simulink model "eomIntegratorChain"  (R2024b)
settings: Solver=ode15s  StartTime=0.0  StopTime=40  MaxStep=0.0001  RelTol=1e-6
values from neighbouring files (symbols this model uses):
  A : value not decoded    [eomParameters.sldd]
  B : value not decoded    [eomParameters.sldd]
  b = 0.1    [eomParameters.sldd]
  C : value not decoded    [eomParameters.sldd]
  D : value not decoded    [eomParameters.sldd]
  d : value not decoded    [eomParameters.sldd]
  E : value not decoded    [eomParameters.sldd]
  F : value not decoded    [eomParameters.sldd]
  H : value not decoded    [eomParameters.sldd]
  I : value not decoded    [eomParameters.sldd]
  J : value not decoded    [eomParameters.sldd]
  K : value not decoded    [eomParameters.sldd]
  L_1 : value not decoded    [eomParameters.sldd]
  mu = 0.4    [eomParameters.sldd]
  mu_r = 0.001    [eomParameters.sldd]
undefined symbols (not defined in the file or in its folder): DiscIntNeverNeededParam
settings Model: DataDictionary=eomParameters.sldd  Creator=nilgunozbulbul  LastModifiedBy=nilgunozbulbul
settings DebuggingCC: SignalInfNanChecking=error

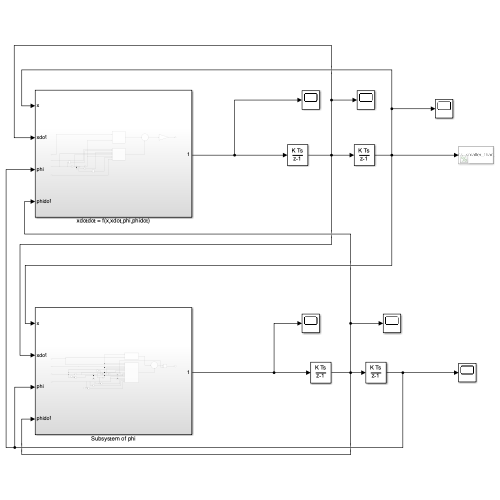
[thumbnail: Simulink's stored preview of the top-level diagram]
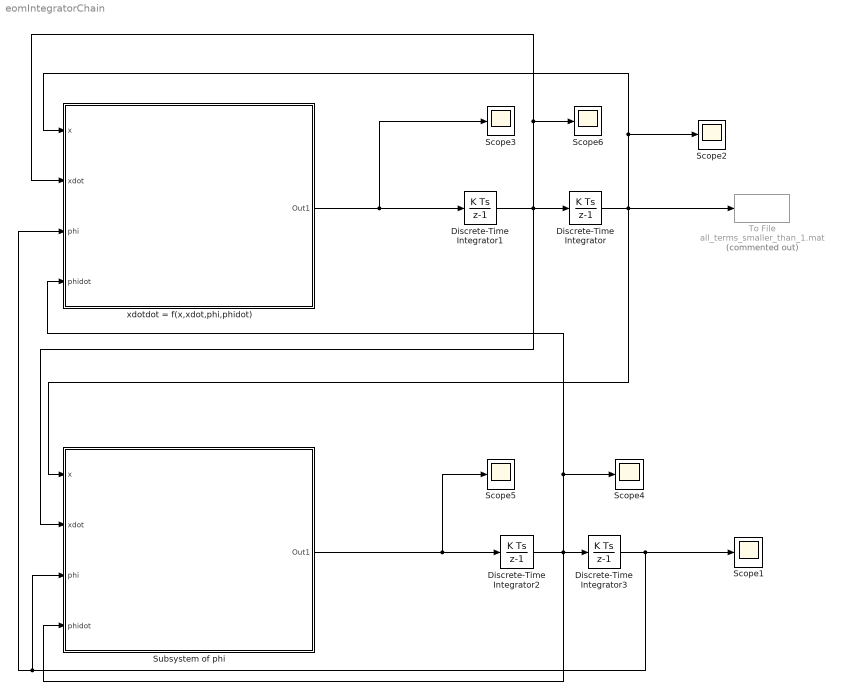
== system eomIntegratorChain ==
  Discrete-Time Integrator : DiscreteIntegrator  InitialCondition=0.05  SampleTime=0.05  UpperSaturationLimit=+100  LowerSaturationLimit=-100  ICPrevOutput=DiscIntNeverNeededParam  ICPrevScaledInput=DiscIntNeverNeededParam
  Discrete-Time Integrator1 : DiscreteIntegrator  SampleTime=0.05  UpperSaturationLimit=0.25  LowerSaturationLimit=-0.25  ICPrevOutput=DiscIntNeverNeededParam  ICPrevScaledInput=DiscIntNeverNeededParam
  Discrete-Time Integrator2 : DiscreteIntegrator  SampleTime=0.05  UpperSaturationLimit=0.9  LowerSaturationLimit=-0.9  ICPrevOutput=DiscIntNeverNeededParam  ICPrevScaledInput=DiscIntNeverNeededParam
  Discrete-Time Integrator3 : DiscreteIntegrator  InitialCondition=0.1  SampleTime=0.05  UpperSaturationLimit=+100  LowerSaturationLimit=-100  ICPrevOutput=DiscIntNeverNeededParam  ICPrevScaledInput=DiscIntNeverNeededParam
  Scope{1..6} (6 alike) : Scope
  Subsystem of phi : Subsystem
  To File : ToFile  Commented=on  Filename=all_terms_smaller_than_1.mat  MatrixName=all_terms_smaller_than_1  SampleTime=0.05
  xdotdot = f(x,xdot,phi,phidot) : Subsystem
  wires:
  Subsystem of phi/1(Out1) -> Discrete-Time Integrator2/1, Scope5/1
  Discrete-Time Integrator2/1 -> Discrete-Time Integrator3/1, xdotdot = f(x,xdot,phi,phidot)/4(phidot), Scope4/1, Subsystem of phi/4(phidot)
  Discrete-Time Integrator3/1 -> xdotdot = f(x,xdot,phi,phidot)/3(phi), Subsystem of phi/3(phi), Scope1/1
  Discrete-Time Integrator1/1 -> Subsystem of phi/2(xdot), Discrete-Time Integrator/1, Scope6/1, xdotdot = f(x,xdot,phi,phidot)/2(xdot)
  xdotdot = f(x,xdot,phi,phidot)/1(Out1) -> Discrete-Time Integrator1/1, Scope3/1
  Discrete-Time Integrator/1 -> Scope2/1, xdotdot = f(x,xdot,phi,phidot)/1(x), To File/1, Subsystem of phi/1(x)

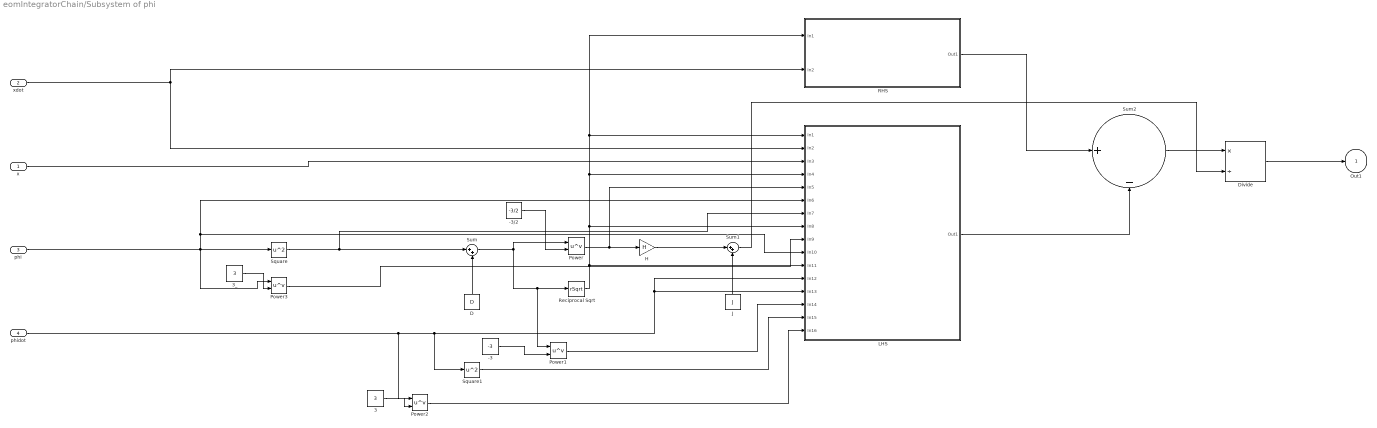
== system eomIntegratorChain/Subsystem of phi ==
  x : Inport
  xdot : Inport  Port=2
  phi : Inport  Port=3
  phidot : Inport  Port=4
  -3 : Constant  Value=-3
  -3/2 : Constant  Value=-3/2
  3 : Constant  Value=3
  3_ : Constant  Value=3
  D : Constant  Value=D
  Divide : Product  Inputs=*/
  H : Gain  Gain=H
  J : Constant  Value=J
  LHS : Subsystem
  Power{,1..3} (4 alike) : Math  Operator=pow
  RHS : Subsystem
  Reciprocal Sqrt : Sqrt  Operator=rSqrt
  Square : Math  Operator=square
  Square1 : Math  Operator=square
  Sum : Sum  Inputs=|++
  Sum1 : Sum  Inputs=|++
  Sum2 : Sum  Inputs=|+-
  Out1 : Outport
  wires:
  Square/1 -> LHS/7(In7), Sum/1
  D/1 -> Sum/2
  Sum/1 -> Power1/1, Reciprocal Sqrt/1, Power/1
  Power/1 -> LHS/5(In5), H/1
  H/1 -> Sum1/1
  J/1 -> Sum1/2
  phidot/1 -> LHS/12(In12), LHS/13(In13), Square1/1, Power2/1
  Divide/1 -> Out1/1
  phi/1 -> LHS/10(In10), LHS/6(In6), Power3/1, Square/1
  xdot/1 -> LHS/2(In2), RHS/2(In2)
  Reciprocal Sqrt/1 -> RHS/1(In1), LHS/1(In1), LHS/4(In4), LHS/8(In8), LHS/11(In11)
  -3/2/1 -> Power/2
  -3/1 -> Power1/2
  3/1 -> Power2/2
  3_/1 -> Power3/2
  x/1 -> LHS/3(In3)
  Power3/1 -> LHS/9(In9)
  Power1/1 -> LHS/14(In14)
  Square1/1 -> LHS/15(In15)
  Power2/1 -> LHS/16(In16)
  LHS/1(Out1) -> Sum2/2
  RHS/1(Out1) -> Sum2/1
  Sum2/1 -> Divide/1
  Sum1/1 -> Divide/2

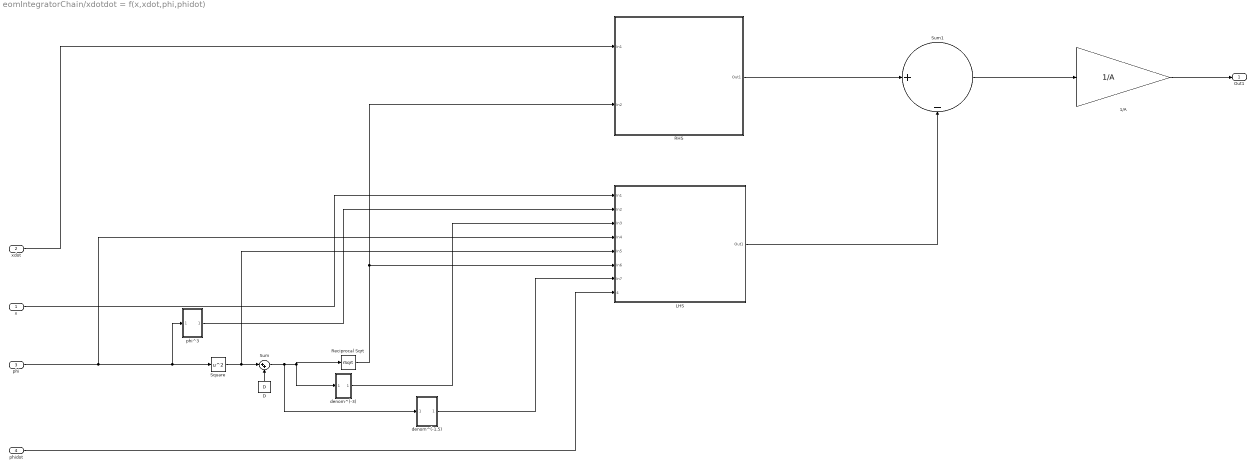
== system eomIntegratorChain/xdotdot = f(x,xdot,phi,phidot) ==
  x : Inport
  xdot : Inport  Port=2
  phi : Inport  Port=3
  phidot : Inport  Port=4
  1/A : Gain  Gain=1/A
  D : Constant  Value=D
  LHS : Subsystem
  RHS : Subsystem
  Reciprocal Sqrt : Sqrt  Operator=rSqrt
  Square : Math  Operator=square
  Sum : Sum  Inputs=|++
  Sum1 : Sum  Inputs=|+-
  denom^(-1.5) : Subsystem
  denom^(-3) : Subsystem
  phi^3 : Subsystem
  Out1 : Outport
  wires:
  phi/1 -> LHS/4(In4), Square/1, phi^3/1(In1)
  Square/1 -> LHS/5(In5), Sum/1
  D/1 -> Sum/2
  Reciprocal Sqrt/1 -> LHS/6(In6), RHS/2(In2)
  Sum/1 -> Reciprocal Sqrt/1, denom^(-3)/1(In1), denom^(-1.5)/1(In1)
  xdot/1 -> RHS/1(In1)
  x/1 -> LHS/1(In1)
  phi^3/1(Out1) -> LHS/2(In2)
  denom^(-3)/1(Out1) -> LHS/3(In3)
  denom^(-1.5)/1(Out1) -> LHS/7(In7)
  phidot/1 -> LHS/8(4)
  RHS/1(Out1) -> Sum1/1
  LHS/1(Out1) -> Sum1/2
  Sum1/1 -> 1/A/1
  1/A/1 -> Out1/1

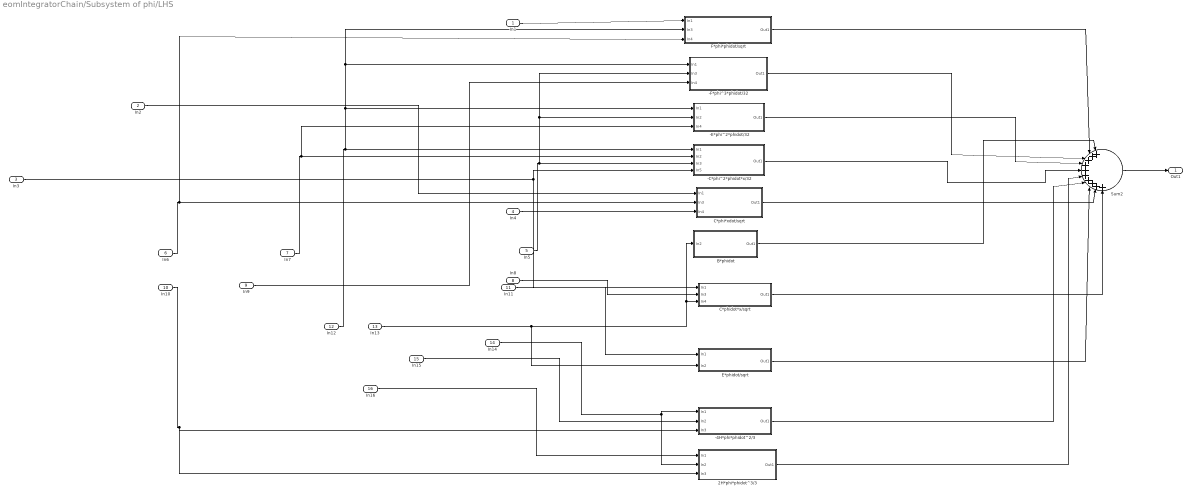
== system eomIntegratorChain/Subsystem of phi/LHS ==
  In1 : Inport
  In2 : Inport  Port=2
  In3 : Inport  Port=3
  In4 : Inport  Port=4
  In5 : Inport  Port=5
  In6 : Inport  Port=6
  In7 : Inport  Port=7
  In8 : Inport  Port=8
  In9 : Inport  Port=9
  In10 : Inport  Port=10
  In11 : Inport  Port=11
  In12 : Inport  Port=12
  In13 : Inport  Port=13
  In14 : Inport  Port=14
  In15 : Inport  Port=15
  In16 : Inport  Port=16
  -4H*phi*phidot^2/3 : Subsystem
  -C*phi^2*phidot*x/32 : Subsystem
  -E*phi^2*phidot/32 : Subsystem
  -F*phi^3*phidot/32 : Subsystem
  2H*phi*phidot^3/3 : Subsystem
  B*phidot : Subsystem
  C*phi*xdot/sqrt : Subsystem
  C*phidot*x/sqrt : Subsystem
  E*phidot/sqrt : Subsystem
  F*phi*phidot/sqrt : Subsystem
  Sum2 : Sum  Inputs=|++++++++++
  Out1 : Outport
  wires:
  C*phidot*x/sqrt/1(Out1) -> Sum2/10
  In9/1 -> -F*phi^3*phidot/32/3(In4)
  In16/1 -> 2H*phi*phidot^3/3/1(In1)
  B*phidot/1(Out1) -> Sum2/1
  In11/1 -> E*phidot/sqrt/1(In1)
  In1/1 -> F*phi*phidot/sqrt/1(In1)
  -C*phi^2*phidot*x/32/1(Out1) -> Sum2/5
  C*phi*xdot/sqrt/1(Out1) -> Sum2/9
  F*phi*phidot/sqrt/1(Out1) -> Sum2/2
  In15/1 -> -4H*phi*phidot^2/3/2(In2)
  2H*phi*phidot^3/3/1(Out1) -> Sum2/6
  In3/1 -> C*phidot*x/sqrt/1(In1), -C*phi^2*phidot*x/32/4(In5)
  In8/1 -> C*phidot*x/sqrt/2(In3)
  In7/1 -> -E*phi^2*phidot/32/3(In4), -C*phi^2*phidot*x/32/2(In2)
  -E*phi^2*phidot/32/1(Out1) -> Sum2/4
  In4/1 -> C*phi*xdot/sqrt/3(In4)
  -F*phi^3*phidot/32/1(Out1) -> Sum2/3
  In13/1 -> E*phidot/sqrt/2(In2), C*phidot*x/sqrt/3(In4), B*phidot/1(In2)
  In14/1 -> 2H*phi*phidot^3/3/2(In2), -4H*phi*phidot^2/3/1(In1)
  In2/1 -> C*phi*xdot/sqrt/1(In1)
  E*phidot/sqrt/1(Out1) -> Sum2/8
  -4H*phi*phidot^2/3/1(Out1) -> Sum2/7
  In5/1 -> -F*phi^3*phidot/32/2(In3), -E*phi^2*phidot/32/2(In2), -C*phi^2*phidot*x/32/3(In3)
  In10/1 -> 2H*phi*phidot^3/3/3(In3), -4H*phi*phidot^2/3/3(In3)
  In6/1 -> F*phi*phidot/sqrt/3(In4), C*phi*xdot/sqrt/2(In3)
  In12/1 -> F*phi*phidot/sqrt/2(In3), -F*phi^3*phidot/32/1(In1), -E*phi^2*phidot/32/1(In1), -C*phi^2*phidot*x/32/1(In1)
  Sum2/1 -> Out1/1

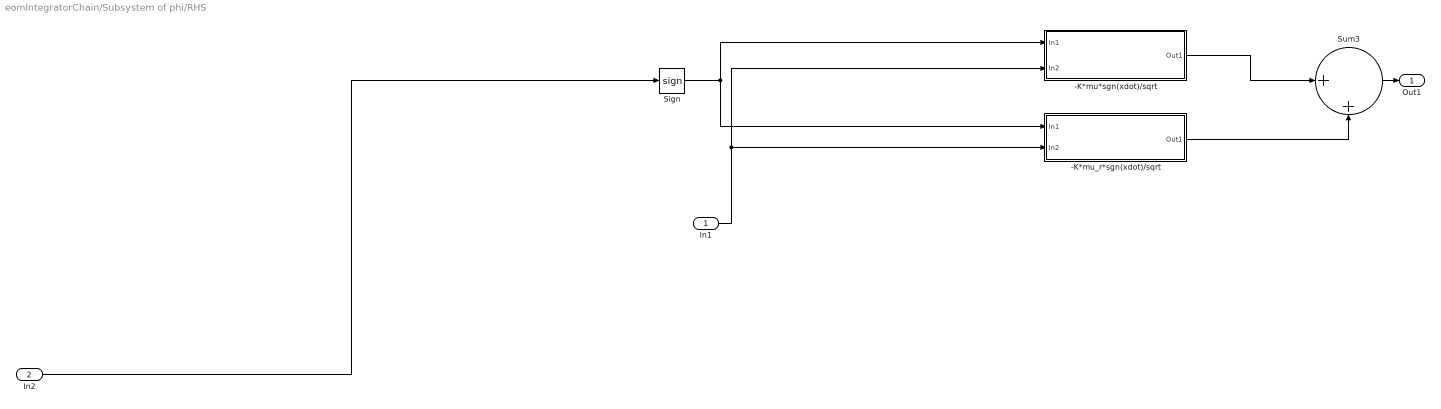
== system eomIntegratorChain/Subsystem of phi/RHS ==
  In1 : Inport
  In2 : Inport  Port=2
  -K*mu*sgn(xdot)/sqrt : Subsystem
  -K*mu_r*sgn(xdot)/sqrt : Subsystem
  Sign : Signum  ZeroCross=off
  Sum3 : Sum  Inputs=|++
  Out1 : Outport
  wires:
  -K*mu_r*sgn(xdot)/sqrt/1(Out1) -> Sum3/2
  In2/1 -> Sign/1
  -K*mu*sgn(xdot)/sqrt/1(Out1) -> Sum3/1
  Sum3/1 -> Out1/1
  In1/1 -> -K*mu*sgn(xdot)/sqrt/2(In2), -K*mu_r*sgn(xdot)/sqrt/2(In2)
  Sign/1 -> -K*mu_r*sgn(xdot)/sqrt/1(In1), -K*mu*sgn(xdot)/sqrt/1(In1)

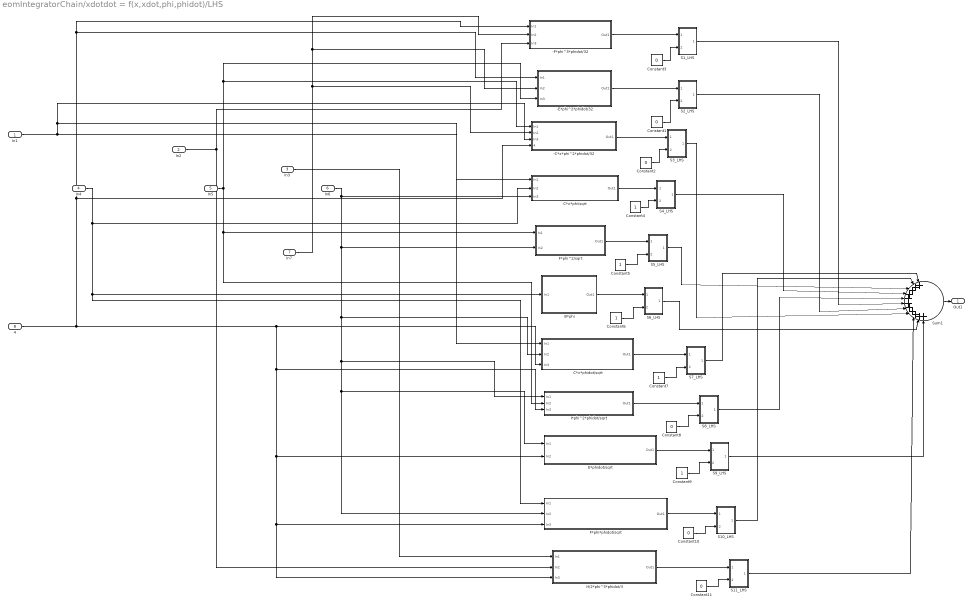
== system eomIntegratorChain/xdotdot = f(x,xdot,phi,phidot)/LHS ==
  In1 : Inport
  In2 : Inport  Port=2
  In3 : Inport  Port=3
  In4 : Inport  Port=4
  In5 : Inport  Port=5
  In6 : Inport  Port=6
  In7 : Inport  Port=7
  4 : Inport  Port=8
  -C*x*phi^2*phidot/32 : Subsystem
  -E*phi^2*phidot/32 : Subsystem
  -F*phi^3*phidot/32 : Subsystem
  B*phi : Subsystem
  C*x*phi/sqrt : Subsystem
  C*x*phidot/sqrt : Subsystem
  Constant{1..3,8,10..11} (6 alike) : Constant  Value=0
  Constant{4..7,9} (5 alike) : Constant
  E*phidot/sqrt : Subsystem
  F*phi*phidot/sqrt : Subsystem
  F*phi^2/sqrt : Subsystem
  H/2*phi^3*phidot/3 : Subsystem
  I*phi^2*phidot/sqrt : Subsystem
  S10_LHS : Subsystem
  S11_LHS : Subsystem
  S1_LHS : Subsystem
  S2_LHS : Subsystem
  S3_LHS : Subsystem
  S4_LHS : Subsystem
  S5_LHS : Subsystem
  S6_LHS : Subsystem
  S7_LHS : Subsystem
  S8_LHS : Subsystem
  S9_LHS : Subsystem
  Sum1 : Sum  Inputs=|+++++++++++
  Out1 : Outport
  wires:
  Sum1/1 -> Out1/1
  In7/1 -> -F*phi^3*phidot/32/2(In2), -E*phi^2*phidot/32/2(In2), -C*x*phi^2*phidot/32/2(In2)
  In5/1 -> F*phi^2/sqrt/1(In1), I*phi^2*phidot/sqrt/2(In2), -E*phi^2*phidot/32/3(In3), -C*x*phi^2*phidot/32/1(In1)
  In2/1 -> H/2*phi^3*phidot/3/2(In2), -F*phi^3*phidot/32/3(In3)
  In1/1 -> C*x*phidot/sqrt/1(In1), -C*x*phi^2*phidot/32/3(In3), C*x*phi/sqrt/1(In1)
  In3/1 -> H/2*phi^3*phidot/3/1(In1)
  In4/1 -> C*x*phi/sqrt/2(In2), F*phi*phidot/sqrt/1(In1), B*phi/1(In1)
  In6/1 -> F*phi^2/sqrt/2(In2), I*phi^2*phidot/sqrt/1(In1), E*phidot/sqrt/1(In1), F*phi*phidot/sqrt/2(In2), C*x*phidot/sqrt/2(In2), C*x*phi/sqrt/3(In3)
  4/1 -> -F*phi^3*phidot/32/1(In1), -E*phi^2*phidot/32/1(In1), -C*x*phi^2*phidot/32/4(4), F*phi*phidot/sqrt/3(In3), H/2*phi^3*phidot/3/3(In3), E*phidot/sqrt/2(In2), I*phi^2*phidot/sqrt/3(In3), C*x*phidot/sqrt/3(In3)
  Constant3/1 -> S1_LHS/2(In2)
  -F*phi^3*phidot/32/1(Out1) -> S1_LHS/1(In1)
  S1_LHS/1(Out1) -> Sum1/6
  Constant1/1 -> S2_LHS/2(In2)
  -E*phi^2*phidot/32/1(Out1) -> S2_LHS/1(In1)
  S2_LHS/1(Out1) -> Sum1/7
  Constant2/1 -> S3_LHS/2(In2)
  -C*x*phi^2*phidot/32/1(Out1) -> S3_LHS/1(In1)
  S3_LHS/1(Out1) -> Sum1/8
  Constant4/1 -> S4_LHS/2(In2)
  C*x*phi/sqrt/1(Out1) -> S4_LHS/1(In1)
  S4_LHS/1(Out1) -> Sum1/4
  Constant5/1 -> S5_LHS/2(In2)
  F*phi^2/sqrt/1(Out1) -> S5_LHS/1(In1)
  S5_LHS/1(Out1) -> Sum1/3
  Constant6/1 -> S6_LHS/2(In2)
  B*phi/1(Out1) -> S6_LHS/1(In1)
  S6_LHS/1(Out1) -> Sum1/10
  Constant7/1 -> S7_LHS/2(In2)
  C*x*phidot/sqrt/1(Out1) -> S7_LHS/1(In1)
  S7_LHS/1(Out1) -> Sum1/1
  Constant8/1 -> S8_LHS/2(In2)
  I*phi^2*phidot/sqrt/1(Out1) -> S8_LHS/1(In1)
  S8_LHS/1(Out1) -> Sum1/5
  Constant9/1 -> S9_LHS/2(In2)
  E*phidot/sqrt/1(Out1) -> S9_LHS/1(In1)
  S9_LHS/1(Out1) -> Sum1/11
  Constant10/1 -> S10_LHS/2(In2)
  F*phi*phidot/sqrt/1(Out1) -> S10_LHS/1(In1)
  S10_LHS/1(Out1) -> Sum1/2
  Constant11/1 -> S11_LHS/2(In2)
  H/2*phi^3*phidot/3/1(Out1) -> S11_LHS/1(In1)
  S11_LHS/1(Out1) -> Sum1/9

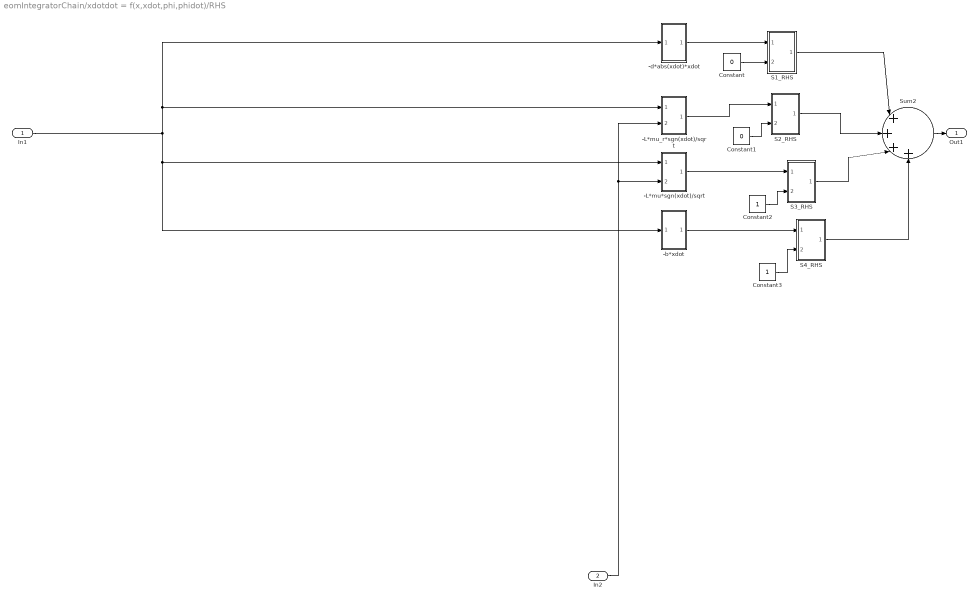
== system eomIntegratorChain/xdotdot = f(x,xdot,phi,phidot)/RHS ==
  In1 : Inport
  In2 : Inport  Port=2
  -L*mu*sgn(xdot)/sqrt : Subsystem
  -L*mu_r*sgn(xdot)/sqrt : Subsystem
  -b*xdot : Subsystem
  -d*abs(xdot)*xdot : Subsystem
  Constant : Constant  Value=0
  Constant1 : Constant  Value=0
  Constant2 : Constant
  Constant3 : Constant
  S1_RHS : Subsystem
  S2_RHS : Subsystem
  S3_RHS : Subsystem
  S4_RHS : Subsystem
  Sum2 : Sum  Inputs=|++++
  Out1 : Outport
  wires:
  Sum2/1 -> Out1/1
  In1/1 -> -d*abs(xdot)*xdot/1(In1), -L*mu_r*sgn(xdot)/sqrt/1(In1), -b*xdot/1(In1), -L*mu*sgn(xdot)/sqrt/1(In1)
  In2/1 -> -L*mu_r*sgn(xdot)/sqrt/2(In2), -L*mu*sgn(xdot)/sqrt/2(In2)
  -d*abs(xdot)*xdot/1(Out1) -> S1_RHS/1(In1)
  Constant/1 -> S1_RHS/2(In2)
  S1_RHS/1(Out1) -> Sum2/1
  -L*mu_r*sgn(xdot)/sqrt/1(Out1) -> S2_RHS/1(In1)
  S2_RHS/1(Out1) -> Sum2/2
  Constant1/1 -> S2_RHS/2(In2)
  Constant2/1 -> S3_RHS/2(In2)
  -L*mu*sgn(xdot)/sqrt/1(Out1) -> S3_RHS/1(In1)
  S3_RHS/1(Out1) -> Sum2/3
  Constant3/1 -> S4_RHS/2(In2)
  -b*xdot/1(Out1) -> S4_RHS/1(In1)
  S4_RHS/1(Out1) -> Sum2/4

== system eomIntegratorChain/xdotdot = f(x,xdot,phi,phidot)/denom^(-1.5) ==
  In1 : Inport
  3/2 : Constant  Value=-1.5
  Power1 : Math  Operator=pow
  Out1 : Outport
  wires:
  In1/1 -> Power1/1
  Power1/1 -> Out1/1
  3/2/1 -> Power1/2

== system eomIntegratorChain/xdotdot = f(x,xdot,phi,phidot)/denom^(-3) ==
  In1 : Inport
  3 : Constant  Value=-3
  Power2 : Math  Operator=pow
  Out1 : Outport
  wires:
  Power2/1 -> Out1/1
  In1/1 -> Power2/1
  3/1 -> Power2/2

== system eomIntegratorChain/xdotdot = f(x,xdot,phi,phidot)/phi^3 ==
  In1 : Inport
  3_ : Constant  Value=3
  Power3 : Math  Operator=pow
  Out1 : Outport
  wires:
  Power3/1 -> Out1/1
  In1/1 -> Power3/1
  3_/1 -> Power3/2

== system eomIntegratorChain/Subsystem of phi/LHS/-4H*phi*phidot^2//3 ==
  In1 : Inport
  In2 : Inport  Port=2
  In3 : Inport  Port=3
  -4H : Gain  Gain=-4*H
  Product7 : Product  Inputs=3
  Out1 : Outport
  wires:
  In3/1 -> Product7/1
  In1/1 -> Product7/2
  Product7/1 -> -4H/1
  In2/1 -> Product7/3
  -4H/1 -> Out1/1

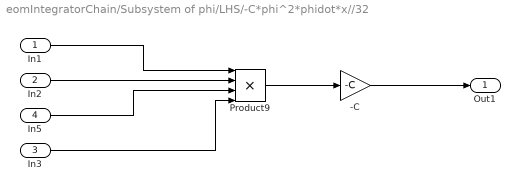
== system eomIntegratorChain/Subsystem of phi/LHS/-C*phi^2*phidot*x//32 ==
  In1 : Inport
  In2 : Inport  Port=2
  In3 : Inport  Port=3
  In5 : Inport  Port=4
  -C : Gain  Gain=-C
  Product9 : Product  Inputs=4
  Out1 : Outport
  wires:
  In2/1 -> Product9/2
  In5/1 -> Product9/3
  In3/1 -> Product9/4
  In1/1 -> Product9/1
  -C/1 -> Out1/1
  Product9/1 -> -C/1

== system eomIntegratorChain/Subsystem of phi/LHS/-E*phi^2*phidot//32 ==
  In1 : Inport
  In2 : Inport  Port=2
  In4 : Inport  Port=3
  -E : Gain  Gain=-E
  Product10 : Product  Inputs=3
  Out1 : Outport
  wires:
  In4/1 -> Product10/2
  In2/1 -> Product10/3
  In1/1 -> Product10/1
  Product10/1 -> -E/1
  -E/1 -> Out1/1

== system eomIntegratorChain/Subsystem of phi/LHS/-F*phi^3*phidot//32 ==
  In1 : Inport
  In3 : Inport  Port=2
  In4 : Inport  Port=3
  -F : Gain  Gain=-F
  Product11 : Product  Inputs=3
  Out1 : Outport
  wires:
  -F/1 -> Out1/1
  In3/1 -> Product11/3
  In4/1 -> Product11/2
  In1/1 -> Product11/1
  Product11/1 -> -F/1

== system eomIntegratorChain/Subsystem of phi/LHS/2H*phi*phidot^3//3 ==
  In1 : Inport
  In2 : Inport  Port=2
  In3 : Inport  Port=3
  2H : Gain  Gain=2*H
  Product8 : Product  Inputs=3
  Out1 : Outport
  wires:
  In2/1 -> Product8/1
  In1/1 -> Product8/3
  Product8/1 -> 2H/1
  In3/1 -> Product8/2
  2H/1 -> Out1/1

== system eomIntegratorChain/Subsystem of phi/LHS/B*phidot ==
  In2 : Inport
  B : Gain  Gain=B
  Out1 : Outport
  wires:
  B/1 -> Out1/1
  In2/1 -> B/1

== system eomIntegratorChain/Subsystem of phi/LHS/C*phi*xdot//sqrt ==
  In1 : Inport
  In3 : Inport  Port=2
  In4 : Inport  Port=3
  C : Gain  Gain=C
  Product3 : Product  Inputs=3
  Out1 : Outport
  wires:
  C/1 -> Out1/1
  In3/1 -> Product3/2
  In4/1 -> Product3/3
  In1/1 -> Product3/1
  Product3/1 -> C/1

== system eomIntegratorChain/Subsystem of phi/LHS/C*phidot*x//sqrt ==
  In1 : Inport
  In3 : Inport  Port=2
  In4 : Inport  Port=3
  C : Gain  Gain=C
  Product : Product  Inputs=3
  Out1 : Outport
  wires:
  C/1 -> Out1/1
  In3/1 -> Product/2
  In4/1 -> Product/3
  In1/1 -> Product/1
  Product/1 -> C/1

== system eomIntegratorChain/Subsystem of phi/LHS/E*phidot//sqrt ==
  In1 : Inport
  In2 : Inport  Port=2
  E : Gain  Gain=E
  Product1 : Product
  Out1 : Outport
  wires:
  E/1 -> Out1/1
  In2/1 -> Product1/2
  In1/1 -> Product1/1
  Product1/1 -> E/1

== system eomIntegratorChain/Subsystem of phi/LHS/F*phi*phidot//sqrt ==
  In1 : Inport
  In3 : Inport  Port=2
  In4 : Inport  Port=3
  F : Gain  Gain=F
  Product12 : Product  Inputs=3
  Out1 : Outport
  wires:
  In3/1 -> Product12/2
  In4/1 -> Product12/1
  F/1 -> Out1/1
  In1/1 -> Product12/3
  Product12/1 -> F/1

== system eomIntegratorChain/Subsystem of phi/RHS/-K*mu*sgn(xdot)//sqrt ==
  In1 : Inport
  In2 : Inport  Port=2
  -K1 : Gain  Gain=-K
  Product14 : Product  Inputs=3
  mu : Constant  Value=mu
  Out1 : Outport
  wires:
  In1/1 -> Product14/2
  In2/1 -> Product14/3
  Product14/1 -> -K1/1
  -K1/1 -> Out1/1
  mu/1 -> Product14/1

== system eomIntegratorChain/Subsystem of phi/RHS/-K*mu_r*sgn(xdot)//sqrt ==
  In1 : Inport
  In2 : Inport  Port=2
  -K : Gain  Gain=-K
  Product13 : Product  Inputs=3
  mu_r : Constant  Value=mu_r
  Out1 : Outport
  wires:
  In1/1 -> Product13/1
  -K/1 -> Out1/1
  Product13/1 -> -K/1
  mu_r/1 -> Product13/3
  In2/1 -> Product13/2

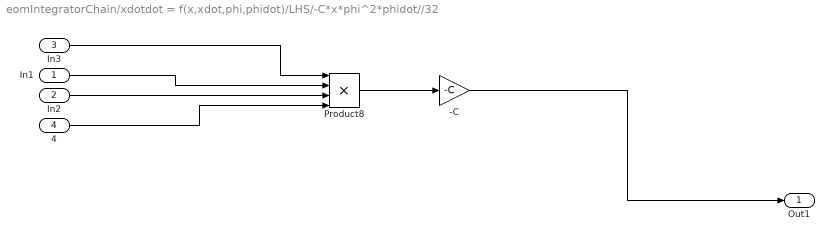
== system eomIntegratorChain/xdotdot = f(x,xdot,phi,phidot)/LHS/-C*x*phi^2*phidot//32 ==
  In1 : Inport
  In2 : Inport  Port=2
  In3 : Inport  Port=3
  4 : Inport  Port=4
  -C : Gain  Gain=-C
  Product8 : Product  Inputs=4
  Out1 : Outport
  wires:
  -C/1 -> Out1/1
  In2/1 -> Product8/3
  In3/1 -> Product8/1
  In1/1 -> Product8/2
  Product8/1 -> -C/1
  4/1 -> Product8/4

== system eomIntegratorChain/xdotdot = f(x,xdot,phi,phidot)/LHS/-E*phi^2*phidot//32 ==
  In1 : Inport
  In2 : Inport  Port=2
  In3 : Inport  Port=3
  -E : Gain  Gain=-E
  Product9 : Product  Inputs=3
  Out1 : Outport
  wires:
  -E/1 -> Out1/1
  In2/1 -> Product9/3
  In1/1 -> Product9/1
  In3/1 -> Product9/2
  Product9/1 -> -E/1

== system eomIntegratorChain/xdotdot = f(x,xdot,phi,phidot)/LHS/-F*phi^3*phidot//32 ==
  In1 : Inport
  In2 : Inport  Port=2
  In3 : Inport  Port=3
  -F : Gain  Gain=-F
  Product10 : Product  Inputs=3
  Out1 : Outport
  wires:
  In3/1 -> Product10/2
  -F/1 -> Out1/1
  In2/1 -> Product10/3
  In1/1 -> Product10/1
  Product10/1 -> -F/1

== system eomIntegratorChain/xdotdot = f(x,xdot,phi,phidot)/LHS/B*phi ==
  In1 : Inport
  B : Gain  Gain=B
  Out1 : Outport
  wires:
  In1/1 -> B/1
  B/1 -> Out1/1

== system eomIntegratorChain/xdotdot = f(x,xdot,phi,phidot)/LHS/C*x*phi//sqrt ==
  In1 : Inport
  In2 : Inport  Port=2
  In3 : Inport  Port=3
  C : Gain  Gain=C
  Product3 : Product  Inputs=3
  Out1 : Outport
  wires:
  In1/1 -> Product3/2
  In3/1 -> Product3/3
  C/1 -> Out1/1
  In2/1 -> Product3/1
  Product3/1 -> C/1

== system eomIntegratorChain/xdotdot = f(x,xdot,phi,phidot)/LHS/C*x*phidot//sqrt ==
  In1 : Inport
  In2 : Inport  Port=2
  In3 : Inport  Port=3
  C : Gain  Gain=C
  Product : Product  Inputs=3
  Out1 : Outport
  wires:
  In3/1 -> Product/3
  In1/1 -> Product/1
  In2/1 -> Product/2
  C/1 -> Out1/1
  Product/1 -> C/1

== system eomIntegratorChain/xdotdot = f(x,xdot,phi,phidot)/LHS/E*phidot//sqrt ==
  In1 : Inport
  In2 : Inport  Port=2
  E : Gain  Gain=E
  Product1 : Product
  Out1 : Outport
  wires:
  In2/1 -> Product1/2
  E/1 -> Out1/1
  In1/1 -> Product1/1
  Product1/1 -> E/1

== system eomIntegratorChain/xdotdot = f(x,xdot,phi,phidot)/LHS/F*phi*phidot//sqrt ==
  In1 : Inport
  In2 : Inport  Port=2
  In3 : Inport  Port=3
  F : Gain  Gain=F
  Product2 : Product  Inputs=3
  Out1 : Outport
  wires:
  F/1 -> Out1/1
  In2/1 -> Product2/2
  In3/1 -> Product2/1
  In1/1 -> Product2/3
  Product2/1 -> F/1

== system eomIntegratorChain/xdotdot = f(x,xdot,phi,phidot)/LHS/F*phi^2//sqrt ==
  In1 : Inport
  In2 : Inport  Port=2
  F : Gain  Gain=F
  Product4 : Product
  Out1 : Outport
  wires:
  F/1 -> Out1/1
  In1/1 -> Product4/2
  In2/1 -> Product4/1
  Product4/1 -> F/1

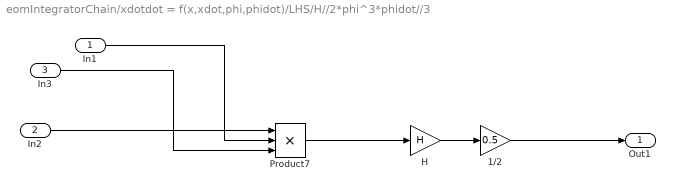
== system eomIntegratorChain/xdotdot = f(x,xdot,phi,phidot)/LHS/H//2*phi^3*phidot//3 ==
  In1 : Inport
  In2 : Inport  Port=2
  In3 : Inport  Port=3
  1/2 : Gain  Gain=0.5
  H : Gain  Gain=H
  Product7 : Product  Inputs=3
  Out1 : Outport
  wires:
  In2/1 -> Product7/1
  In1/1 -> Product7/2
  In3/1 -> Product7/3
  Product7/1 -> H/1
  1/2/1 -> Out1/1
  H/1 -> 1/2/1

== system eomIntegratorChain/xdotdot = f(x,xdot,phi,phidot)/LHS/I*phi^2*phidot//sqrt ==
  In1 : Inport
  In2 : Inport  Port=2
  In3 : Inport  Port=3
  I : Gain  Gain=I
  Product11 : Product  Inputs=3
  Out1 : Outport
  wires:
  I/1 -> Out1/1
  In3/1 -> Product11/3
  In2/1 -> Product11/2
  In1/1 -> Product11/1
  Product11/1 -> I/1

== system eomIntegratorChain/xdotdot = f(x,xdot,phi,phidot)/LHS/S10_LHS ==
  In1 : Inport
  In2 : Inport  Port=2
  Constant1 : Constant  Value=0
  Switch : Switch  Criteria=u2 ~= 0  SaturateOnIntegerOverflow=off  InputSameDT=off
  Out1 : Outport
  wires:
  In1/1 -> Switch/1
  Switch/1 -> Out1/1
  In2/1 -> Switch/2
  Constant1/1 -> Switch/3

== system eomIntegratorChain/xdotdot = f(x,xdot,phi,phidot)/LHS/S11_LHS ==
  In1 : Inport
  In2 : Inport  Port=2
  Constant1 : Constant  Value=0
  Switch : Switch  Criteria=u2 ~= 0  SaturateOnIntegerOverflow=off  InputSameDT=off
  Out1 : Outport
  wires:
  In1/1 -> Switch/1
  Switch/1 -> Out1/1
  In2/1 -> Switch/2
  Constant1/1 -> Switch/3

== system eomIntegratorChain/xdotdot = f(x,xdot,phi,phidot)/LHS/S1_LHS ==
  In1 : Inport
  In2 : Inport  Port=2
  Constant1 : Constant  Value=0
  Switch : Switch  Criteria=u2 ~= 0  SaturateOnIntegerOverflow=off  InputSameDT=off
  Out1 : Outport
  wires:
  In1/1 -> Switch/1
  Switch/1 -> Out1/1
  In2/1 -> Switch/2
  Constant1/1 -> Switch/3

== system eomIntegratorChain/xdotdot = f(x,xdot,phi,phidot)/LHS/S2_LHS ==
  In1 : Inport
  In2 : Inport  Port=2
  Constant1 : Constant  Value=0
  Switch : Switch  Criteria=u2 ~= 0  SaturateOnIntegerOverflow=off  InputSameDT=off
  Out1 : Outport
  wires:
  In1/1 -> Switch/1
  Switch/1 -> Out1/1
  In2/1 -> Switch/2
  Constant1/1 -> Switch/3

== system eomIntegratorChain/xdotdot = f(x,xdot,phi,phidot)/LHS/S3_LHS ==
  In1 : Inport
  In2 : Inport  Port=2
  Constant1 : Constant  Value=0
  Switch : Switch  Criteria=u2 ~= 0  SaturateOnIntegerOverflow=off  InputSameDT=off
  Out1 : Outport
  wires:
  In1/1 -> Switch/1
  Switch/1 -> Out1/1
  In2/1 -> Switch/2
  Constant1/1 -> Switch/3

== system eomIntegratorChain/xdotdot = f(x,xdot,phi,phidot)/LHS/S4_LHS ==
  In1 : Inport
  In2 : Inport  Port=2
  Constant1 : Constant  Value=0
  Switch : Switch  Criteria=u2 ~= 0  SaturateOnIntegerOverflow=off  InputSameDT=off
  Out1 : Outport
  wires:
  In1/1 -> Switch/1
  Switch/1 -> Out1/1
  In2/1 -> Switch/2
  Constant1/1 -> Switch/3

== system eomIntegratorChain/xdotdot = f(x,xdot,phi,phidot)/LHS/S5_LHS ==
  In1 : Inport
  In2 : Inport  Port=2
  Constant1 : Constant  Value=0
  Switch : Switch  Criteria=u2 ~= 0  SaturateOnIntegerOverflow=off  InputSameDT=off
  Out1 : Outport
  wires:
  In1/1 -> Switch/1
  Switch/1 -> Out1/1
  In2/1 -> Switch/2
  Constant1/1 -> Switch/3

== system eomIntegratorChain/xdotdot = f(x,xdot,phi,phidot)/LHS/S6_LHS ==
  In1 : Inport
  In2 : Inport  Port=2
  Constant1 : Constant  Value=0
  Switch : Switch  Criteria=u2 ~= 0  SaturateOnIntegerOverflow=off  InputSameDT=off
  Out1 : Outport
  wires:
  In1/1 -> Switch/1
  Switch/1 -> Out1/1
  In2/1 -> Switch/2
  Constant1/1 -> Switch/3

== system eomIntegratorChain/xdotdot = f(x,xdot,phi,phidot)/LHS/S7_LHS ==
  In1 : Inport
  In2 : Inport  Port=2
  Constant1 : Constant  Value=0
  Switch : Switch  Criteria=u2 ~= 0  SaturateOnIntegerOverflow=off  InputSameDT=off
  Out1 : Outport
  wires:
  In1/1 -> Switch/1
  Switch/1 -> Out1/1
  In2/1 -> Switch/2
  Constant1/1 -> Switch/3

== system eomIntegratorChain/xdotdot = f(x,xdot,phi,phidot)/LHS/S8_LHS ==
  In1 : Inport
  In2 : Inport  Port=2
  Constant1 : Constant  Value=0
  Switch : Switch  Criteria=u2 ~= 0  SaturateOnIntegerOverflow=off  InputSameDT=off
  Out1 : Outport
  wires:
  In1/1 -> Switch/1
  Switch/1 -> Out1/1
  In2/1 -> Switch/2
  Constant1/1 -> Switch/3

== system eomIntegratorChain/xdotdot = f(x,xdot,phi,phidot)/LHS/S9_LHS ==
  In1 : Inport
  In2 : Inport  Port=2
  Constant1 : Constant  Value=0
  Switch : Switch  Criteria=u2 ~= 0  SaturateOnIntegerOverflow=off  InputSameDT=off
  Out1 : Outport
  wires:
  In1/1 -> Switch/1
  Switch/1 -> Out1/1
  In2/1 -> Switch/2
  Constant1/1 -> Switch/3

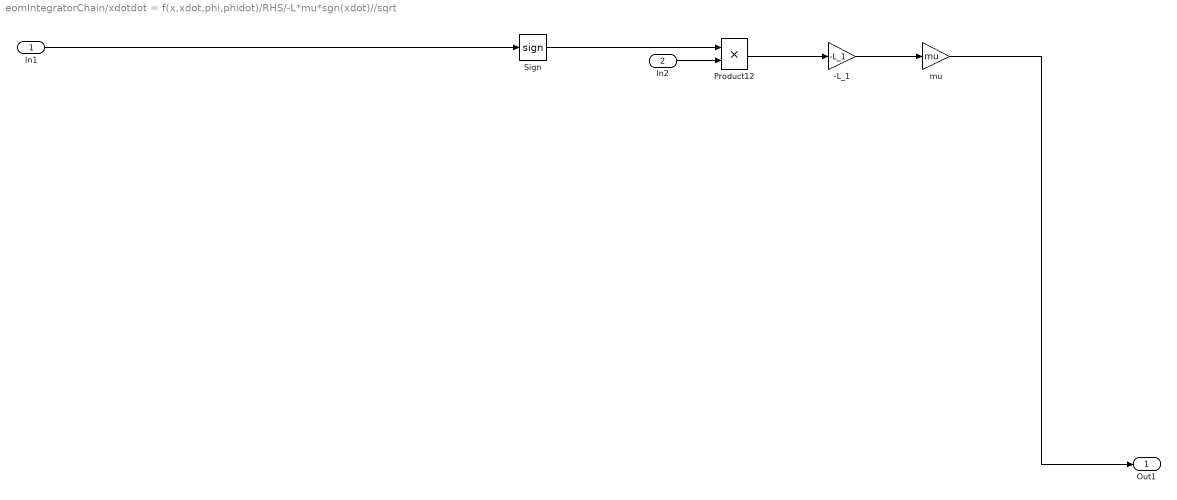
== system eomIntegratorChain/xdotdot = f(x,xdot,phi,phidot)/RHS/-L*mu*sgn(xdot)//sqrt ==
  In1 : Inport
  In2 : Inport  Port=2
  -L_1 : Gain  Gain=-L_1
  Product12 : Product
  Sign : Signum  ZeroCross=off
  mu : Gain  Gain=mu
  Out1 : Outport
  wires:
  In2/1 -> Product12/2
  Sign/1 -> Product12/1
  In1/1 -> Sign/1
  mu/1 -> Out1/1
  Product12/1 -> -L_1/1
  -L_1/1 -> mu/1

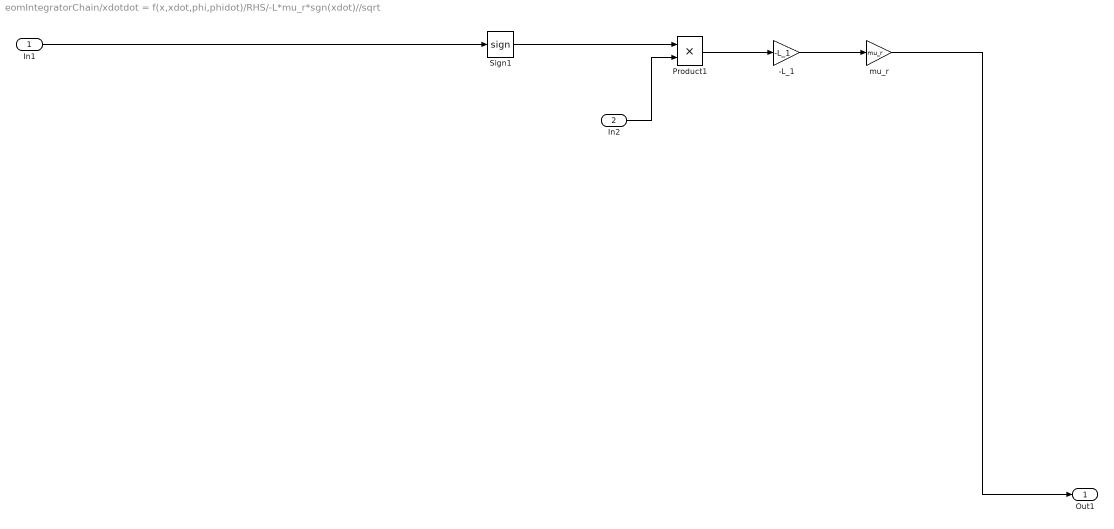
== system eomIntegratorChain/xdotdot = f(x,xdot,phi,phidot)/RHS/-L*mu_r*sgn(xdot)//sqrt ==
  In1 : Inport
  In2 : Inport  Port=2
  -L_1 : Gain  Gain=-L_1
  Product1 : Product
  Sign1 : Signum  ZeroCross=off
  mu_r : Gain  Gain=mu_r
  Out1 : Outport
  wires:
  Product1/1 -> -L_1/1
  -L_1/1 -> mu_r/1
  Sign1/1 -> Product1/1
  In1/1 -> Sign1/1
  In2/1 -> Product1/2
  mu_r/1 -> Out1/1

== system eomIntegratorChain/xdotdot = f(x,xdot,phi,phidot)/RHS/-b*xdot ==
  In1 : Inport
  -b : Gain  Gain=-b
  Out1 : Outport
  wires:
  In1/1 -> -b/1
  -b/1 -> Out1/1

== system eomIntegratorChain/xdotdot = f(x,xdot,phi,phidot)/RHS/-d*abs(xdot)*xdot ==
  In1 : Inport
  -d : Gain  Gain=-d
  Abs : Abs  ZeroCross=off  SaturateOnIntegerOverflow=off
  Product13 : Product
  Scope : Scope
  Scope1 : Scope
  Out1 : Outport
  wires:
  Product13/1 -> Scope1/1, -d/1
  In1/1 -> Scope/1, Product13/1, Abs/1
  -d/1 -> Out1/1
  Abs/1 -> Product13/2

== system eomIntegratorChain/xdotdot = f(x,xdot,phi,phidot)/RHS/S1_RHS ==
  In1 : Inport
  In2 : Inport  Port=2
  Constant1 : Constant  Value=0
  Switch : Switch  Criteria=u2 ~= 0  SaturateOnIntegerOverflow=off  InputSameDT=off
  Out1 : Outport
  wires:
  In1/1 -> Switch/1
  Switch/1 -> Out1/1
  In2/1 -> Switch/2
  Constant1/1 -> Switch/3

== system eomIntegratorChain/xdotdot = f(x,xdot,phi,phidot)/RHS/S2_RHS ==
  In1 : Inport
  In2 : Inport  Port=2
  Constant1 : Constant  Value=0
  Switch : Switch  Criteria=u2 ~= 0  SaturateOnIntegerOverflow=off  InputSameDT=off
  Out1 : Outport
  wires:
  In1/1 -> Switch/1
  Switch/1 -> Out1/1
  In2/1 -> Switch/2
  Constant1/1 -> Switch/3

== system eomIntegratorChain/xdotdot = f(x,xdot,phi,phidot)/RHS/S3_RHS ==
  In1 : Inport
  In2 : Inport  Port=2
  Constant1 : Constant  Value=0
  Switch : Switch  Criteria=u2 ~= 0  SaturateOnIntegerOverflow=off  InputSameDT=off
  Out1 : Outport
  wires:
  In1/1 -> Switch/1
  Switch/1 -> Out1/1
  In2/1 -> Switch/2
  Constant1/1 -> Switch/3

== system eomIntegratorChain/xdotdot = f(x,xdot,phi,phidot)/RHS/S4_RHS ==
  In1 : Inport
  In2 : Inport  Port=2
  Constant1 : Constant  Value=0
  Switch : Switch  Criteria=u2 ~= 0  SaturateOnIntegerOverflow=off  InputSameDT=off
  Out1 : Outport
  wires:
  In1/1 -> Switch/1
  Switch/1 -> Out1/1
  In2/1 -> Switch/2
  Constant1/1 -> Switch/3
